simulink model "qpsk_rc"  (R2018b)
settings: Solver=VariableStepDiscrete  StartTime=0.0  StopTime=200  RelTol=1e-3  EnableMultiTasking=on
libraries: commdigbbndpm3 x2, commfilt2 x2, commchan3 x1, commsink2 x1, commrandsrc3 x1
CloseFcn:
  | clear phnoiseSigsOut
  | 
  | % Close BER figure, if it exists
  | if exist('hPhaseNoise256QAM')  % figure has been created
  |     if ishandle(hPhaseNoise256QAM)  % figure still exists
  |         close(hPhaseNoise256QAM)
  |     end
  |     clear hPhaseNoise256QAM
  | end
Description:
  | Phase Noise Effects in 256-QAM
  | 
  | This model shows the effect of a receiver's phase noise on 256-ary quadrature amplitude modulation (QAM).
settings Model: ExtModeAutoUpdateStatusClock=off  Creator=The MathWorks, Inc.  LastModifiedBy=rka
settings SolverCC: InsertRTBMode=Auto
settings DataIOCC: LimitDataPoints=on  SaveFormat=Array  SaveOutput=off  SaveTime=off  SignalLoggingName=phnoiseSigsOut
settings OptimizationCC: BlockReduction=off  BooleanDataType=off  ExpressionDepthLimit=2147483647  InitFltsAndDblsToZero=on  EfficientMapNaN2IntZero=off  LifeSpan=inf  BufferReusableBoundary=off
settings DebuggingCC: SaveWithParameterizedLinksMsg=none  UnderspecifiedInitializationDetection=Classic  MergeDetectMultiDrivingBlocksExec=none  CheckExecutionContextPreStartOutputMsg=on  CheckExecutionContextRuntimeOutputMsg=on  SignalResolutionControl=TryResolveAllWithWarning  InheritedTsInSrcMsg=none  MultiTaskDSMMsg=warning  MultiTaskCondExecSysMsg=none  SigSpecEnsureSampleTimeMsg=none  ParameterPrecisionLossMsg=none  FcnCallInpInsideContextMsg=warning  BusObjectLabelMismatch=none  StateNameClashWarn=warning  SFUnexpectedBacktrackingDiag=warning  SFNoUnconditionalDefaultTransitionDiag=warning  SFExecutionAtInitializationDiag=none
settings HardwareCC: ProdBitPerPointer=32  ProdBitPerSizeT=32  ProdBitPerPtrDiffT=32  ProdLargestAtomicFloat=None  ProdIntDivRoundTo=Undefined  ProdEndianess=Unspecified  ProdWordSize=32  ProdHWDeviceType=32-bit Generic  TargetUnknown=on
settings ModelReferenceCC: UpdateModelReferenceTargets=IfOutOfDate  PropagateSignalLabelsOutOfModel=off
settings SFSimCC: SimUseLocalCustomCode=off
settings RTWCC: RTWUseLocalCustomCode=off
settings CodeAppCC: StateflowObjectComments=on
settings GRTTargetCC: TargetFcnLib=ansi_tfl_tmw.mat  TargetLangStandard=C89/C90 (ANSI)  GeneratePreprocessorConditionals=Disable all  CombineOutputUpdateFcns=off  GRTInterface=on
settings ConfigComp: CovMetricSettings=dw  CovHtmlReporting=on  CovSaveCumulativeToWorkspaceVar=on  CovSaveSingleToWorkspaceVar=on  CovExternalEMLEnable=off  CovSFcnEnable=off

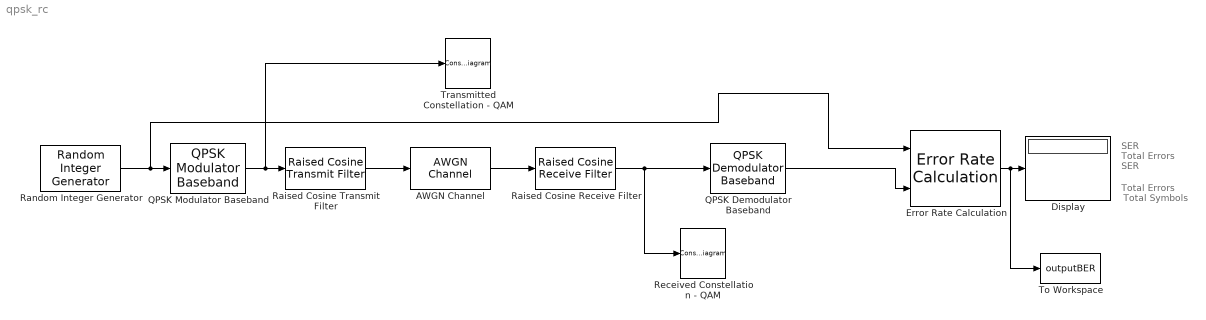
== system qpsk_rc ==
  note: SER
  note: Total Errors
  note: SER
  note: Total Errors
  note: Total Symbols
  AWGN Channel : commchan3/AWGN Channel  InputProcessing=Columns as channels (frame based)  seed=54321  noiseMode="Signal to noise ratio  (SNR)"  EbNodB=50  EsNodB=10  SNRdB=15  bitsPerSym=6  Ps=1  Tsym=1  variance=1
      settings: SourceProductName=Communications Toolbox
  Display : Display
  Error Rate Calculation : commsink2/Error Rate Calculation  N=6  st_delay=0  cp_mode=Entire frame  subframe=[]  PMode=Port  WsName=ErrorVec  RsMode2=off  stop=off  numErr=100  maxBits=1e6
      settings: SourceProductName=Communications Toolbox
  QPSK Demodulator Baseband : commdigbbndpm3/QPSK Demodulator Baseband  OutType=Integer  DecType=Hard decision  VarSource=Dialog  Variance=1  Dec=Gray  Ph=pi/4  outDtype1=Inherit via internal rule  outDtype2=Inherit via internal rule  derotateFactorWordLen=16  derotateFactorDataTypeStr=Inherit: Same word length as input  derotateFactorLastDataTypeStr=Inherit: Same word length as input
  QPSK Modulator Baseband : commdigbbndpm3/QPSK Modulator Baseband  InType=Integer  Enc=Gray  Ph=pi/4  outDtype=double  outWordLen=16  outUDDataType=sfix(16)  outFracLenMode=Best precision  outFracLen=15  outDataTypeStr=double  outLastDataTypeStr=double
  Raised Cosine Receive Filter : commfilt2/Raised Cosine Receive Filter  filtType=Normal  R=0.2  filtSpan=2*3  N=8  downFactor=8  downOffset=0  filterGain=1  InputProcessing=Columns as channels (frame based)  RateOptions=Enforce single-rate processing  framing=Mute  checkCoeff=off  variableName=rcRxFilt  currentFiltSpan=2*3  D=(2*3)/2  inputOffset=0  sampMode=Mute  saveAsFlag=0  rateMode=Downsampling  checkGain=Normalized  launchFVT=on  roundingMode=Floor  overflowMode=off  coeffDataTypeStr=Inherit: Same word length as input  coeffMin=[]  coeffMax=[]  coeffLastDataTypeStr=Inherit: Same word length as input  accumDataTypeStr=Inherit: Same as product output  accumLastDataTypeStr=Inherit: Same as product output  outputDataTypeStr=Inherit: Same as accumulator  outputMin=[]  outputMax=[]  outputLastDataTypeStr=Inherit: Same as accumulator
  Raised Cosine Transmit Filter : commfilt2/Raised Cosine Transmit Filter  filtType=Normal  R=0.2  filtSpan=2*3  N=8  filterGain=1  InputProcessing=Columns as channels (frame based)  RateOptions=Enforce single-rate processing  framing=Mute  checkCoeff=off  variableName=rcTxFilt  checkGain=Normalized  sampMode=Mute  saveAsFlag=0  currentFiltSpan=2*3  D=(2*3)/2  launchFVT=on  roundingMode=Floor  overflowMode=off  coeffDataTypeStr=Inherit: Same word length as input  coeffMin=[]  coeffMax=[]  coeffLastDataTypeStr=Inherit: Same word length as input  outputDataTypeStr=Inherit: Same as accumulator  outputMin=[]  outputMax=[]  outputLastDataTypeStr=Inherit: Same as accumulator
  Random Integer Generator : commrandsrc3/Random Integer Generator  SetSize=4  SeedSource=Auto  Seed=0  SampleTime=1  SamplesPerFrame=1  OutputDataType=uint8  SimulateUsing=Interpreted execution
  Received Constellation - QAM : ConstellationDiagram  Tag=ScatterPlot
  To Workspace : ToWorkspace  VariableName=outputBER  SampleTime=-1
      settings: Decimation=3
  Transmitted Constellation - QAM : ConstellationDiagram  Tag=ScatterPlot
  wires:
  Error Rate Calculation/1 -> To Workspace/1, Display/1
  AWGN Channel/1 -> Raised Cosine Receive Filter/1
  QPSK Modulator Baseband/1 -> Transmitted Constellation - QAM/1, Raised Cosine Transmit Filter/1
  Raised Cosine Transmit Filter/1 -> AWGN Channel/1
  Raised Cosine Receive Filter/1 -> QPSK Demodulator Baseband/1, Received Constellation - QAM/1
  QPSK Demodulator Baseband/1 -> Error Rate Calculation/2
  Random Integer Generator/1 -> QPSK Modulator Baseband/1, Error Rate Calculation/1
